simulink model "robotarm_A11"  (R2018b)
settings: Solver=FixedStepAuto  StartTime=0.0  StopTime=options.T_train  RelTol=1e-3  AbsTol=1e-6
undefined symbols (not defined in the file or in its folder): options
libraries: neural x132, simulink x2
(part 4 of 6)

== system robotarm_A11/NN/Layer 3/Delays 1 ==
  "p{3}" : Inport  PortDimensions=30
      mask Display: e = 0.06;c1 = [120 230 180]/255;c2 = ([120 230 180]+0)/(256+128);c3 = ([120 230 180]+128)/(256+128);patch([0 1 1 0],[0 0 1 1],c1);patch([0 1 1 1-e 1-e 0+e],[0 0 1 1-e 0+e 0+e],c2);patch([0 0 1 1-e 0+e 0+e],[0 1 1 1-e 1-e 0+e],c3);plot([0 1 1 0 0],[0 0 1 1 0]);
  mux : Mux  Inputs=1
      mask Display: e = 0.06;c1 = [120 150 230]/255;c2 = ([120 150 230]+0)/383;c3 = ([120 150 230]+128)/383;patch([0 1 1 0],[0 0 1 1],c1);patch([0 1 1 1-e 1-e 0+e],[0 0 1 1-e 0+e 0+e],c2);patch([0 0 1 1-e 0+e 0+e],[0 1 1 1-e 1-e 0+e],c3);plot([0 1 1 0 0],[0 0 1 1 0]);disp('Mux')
  "pd{3,2}" : Outport
      mask Display: e = 0.06;c1 = [120 230 180]/255;c2 = ([120 230 180]+0)/(256+128);c3 = ([120 230 180]+128)/(256+128);patch([0 1 1 0],[0 0 1 1],c1);patch([0 1 1 1-e 1-e 0+e],[0 0 1 1-e 0+e 0+e],c2);patch([0 0 1 1-e 0+e 0+e],[0 1 1 1-e 1-e 0+e],c3);plot([0 1 1 0 0],[0 0 1 1 0]);
  wires:
  "p{3}"/1 -> mux/1
  mux/1 -> "pd{3,2}"/1

== system robotarm_A11/NN/Layer 3/LW{3,2} ==
  "ad{3,2}" : Inport  PortDimensions=30
      mask Display: e = 0.06;c1 = [120 230 180]/255;c2 = ([120 230 180]+0)/(256+128);c3 = ([120 230 180]+128)/(256+128);patch([0 1 1 0],[0 0 1 1],c1);patch([0 1 1 1-e 1-e 0+e],[0 0 1 1-e 0+e 0+e],c2);patch([0 0 1 1-e 0+e 0+e],[0 1 1 1-e 1-e 0+e],c3);plot([0 1 1 0 0],[0 0 1 1 0]);
  "IW{3,2}(1,:)'" : Constant  Value=[0.07511090421461637245403863971660030074417591094970703125;-0.256099043433060113983401606674306094646453857421875;0.081996461567937439784969910760992206633090972900390625;-0.14973516379113960272917438487638719379901885986328125;0.5148961449988653793496951038832776248455047607421875;0.01324189378345717350848875781821334385313093662261962890625;0.2272209721687915850996120070703909732401371002197265625;-0.2208186824312869112052482023500488139688968658447265625;0.65756683071975541299281076135230250656604766845703125;-0.22237646509733133282082917503430508077144622802734375;-0.3308957162516181771394485622295178472995758056640625;0.637401045576047931007224178756587207317352294921875;0.667089213297717975592604489065706729888916015625;0.497075395905719308320414029367384500801563262939453125;-0.1445442468661915225158764997104299254715442657470703125;-0.336243110161506819633103759770165197551250457763671875;-0.65568518383315710362779782371944747865200042724609375;-0.6382390498773180542713134855148382484912872314453125;-0.44979178921980411676173616797314025461673736572265625;-0.2575443668624275428413739064126275479793548583984375;0.251838451386020290012623945585801266133785247802734375;0.84864546013635833165977828684845007956027984619140625;-0.31882372388745905400497804293991066515445709228515625;-0.27920298783133612463558392846607603132724761962890625;0.81251359569967795959399836647207848727703094482421875;-0.445650703236170731003085165866650640964508056640625;0.12363838330791576680667276377789676189422607421875;0.37180610815353876130728849602746777236461639404296875;-0.239048902638888172145215094133163802325725555419921875;0.06162269083689660142955091259864275343716144561767578125]
      mask Display: e = 0.06;c1 = [120 150 230]/255;c2 = ([120 150 230]+0)/383;c3 = ([120 150 230]+128)/383;patch([0 1 1 0],[0 0 1 1],c1);patch([0 1 1 1-e 1-e 0+e],[0 0 1 1-e 0+e 0+e],c2);patch([0 0 1 1-e 0+e 0+e],[0 1 1 1-e 1-e 0+e],c3);plot([0 1 1 0 0],[0 0 1 1 0]);disp('weights');
  Mux : Mux  Inputs=1
      mask Display: e = 0.06;c1 = [120 150 230]/255;c2 = ([120 150 230]+0)/383;c3 = ([120 150 230]+128)/383;patch([0 1 1 0],[0 0 1 1],c1);patch([0 1 1 1-e 1-e 0+e],[0 0 1 1-e 0+e 0+e],c2);patch([0 0 1 1-e 0+e 0+e],[0 1 1 1-e 1-e 0+e],c3);plot([0 1 1 0 0],[0 0 1 1 0]);disp('Mux');
  dotprod1 : neural/Weight Functions/dotprod
  "lz{3,2}" : Outport
      mask Display: e = 0.06;c1 = [120 230 180]/255;c2 = ([120 230 180]+0)/(256+128);c3 = ([120 230 180]+128)/(256+128);patch([0 1 1 0],[0 0 1 1],c1);patch([0 1 1 1-e 1-e 0+e],[0 0 1 1-e 0+e 0+e],c2);patch([0 0 1 1-e 0+e 0+e],[0 1 1 1-e 1-e 0+e],c3);plot([0 1 1 0 0],[0 0 1 1 0]);
  wires:
  "IW{3,2}(1,:)'"/1 -> dotprod1/1
  "ad{3,2}"/1 -> dotprod1/2
  dotprod1/1 -> Mux/1
  Mux/1 -> "lz{3,2}"/1

== system robotarm_A11/NN_cex_1/Layer 1/Delays 1 ==
  "p{1}" : Inport  PortDimensions=10
      mask Display: e = 0.06;c1 = [120 230 180]/255;c2 = ([120 230 180]+0)/(256+128);c3 = ([120 230 180]+128)/(256+128);patch([0 1 1 0],[0 0 1 1],c1);patch([0 1 1 1-e 1-e 0+e],[0 0 1 1-e 0+e 0+e],c2);patch([0 0 1 1-e 0+e 0+e],[0 1 1 1-e 1-e 0+e],c3);plot([0 1 1 0 0],[0 0 1 1 0]);
  mux : Mux  Inputs=1
      mask Display: e = 0.06;c1 = [120 150 230]/255;c2 = ([120 150 230]+0)/383;c3 = ([120 150 230]+128)/383;patch([0 1 1 0],[0 0 1 1],c1);patch([0 1 1 1-e 1-e 0+e],[0 0 1 1-e 0+e 0+e],c2);patch([0 0 1 1-e 0+e 0+e],[0 1 1 1-e 1-e 0+e],c3);plot([0 1 1 0 0],[0 0 1 1 0]);disp('Mux')
  "pd{1,1}" : Outport
      mask Display: e = 0.06;c1 = [120 230 180]/255;c2 = ([120 230 180]+0)/(256+128);c3 = ([120 230 180]+128)/(256+128);patch([0 1 1 0],[0 0 1 1],c1);patch([0 1 1 1-e 1-e 0+e],[0 0 1 1-e 0+e 0+e],c2);patch([0 0 1 1-e 0+e 0+e],[0 1 1 1-e 1-e 0+e],c3);plot([0 1 1 0 0],[0 0 1 1 0]);
  wires:
  "p{1}"/1 -> mux/1
  mux/1 -> "pd{1,1}"/1

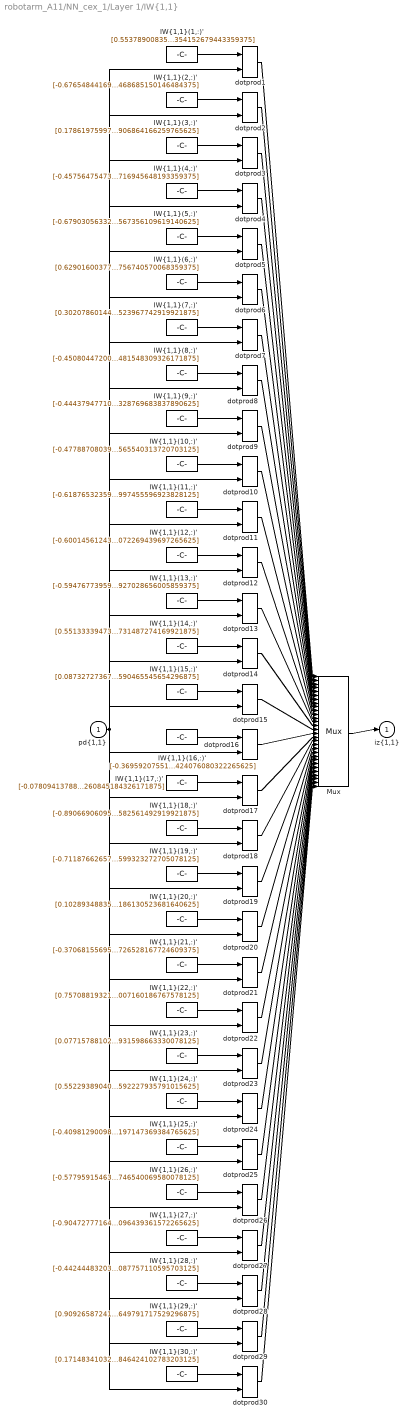
== system robotarm_A11/NN_cex_1/Layer 1/IW{1,1} ==
  "pd{1,1}" : Inport  PortDimensions=10
      mask Display: e = 0.06;c1 = [120 230 180]/255;c2 = ([120 230 180]+0)/(256+128);c3 = ([120 230 180]+128)/(256+128);patch([0 1 1 0],[0 0 1 1],c1);patch([0 1 1 1-e 1-e 0+e],[0 0 1 1-e 0+e 0+e],c2);patch([0 0 1 1-e 0+e 0+e],[0 1 1 1-e 1-e 0+e],c3);plot([0 1 1 0 0],[0 0 1 1 0]);
  "IW{1,1}(1,:)'" : Constant  Value=[0.55378900835415312275955557197448797523975372314453125;-0.40002833313486885202792109339497983455657958984375;0.51972210734784318741930064788903109729290008544921875;0.035441252661289439351843810754871810786426067352294921875;0.58851130139368124094545464686234481632709503173828125;0.373001312883801616759882335827569477260112762451171875;0.1968531470949289874372567510363296605646610260009765625;0.38544814076508793210251724303816445171833038330078125;0.52673681147124951085203292677761055529117584228515625;-0.76855654247942906120982797801843844354152679443359375]
      mask Display: e = 0.06;c1 = [120 150 230]/255;c2 = ([120 150 230]+0)/383;c3 = ([120 150 230]+128)/383;patch([0 1 1 0],[0 0 1 1],c1);patch([0 1 1 1-e 1-e 0+e],[0 0 1 1-e 0+e 0+e],c2);patch([0 0 1 1-e 0+e 0+e],[0 1 1 1-e 1-e 0+e],c3);plot([0 1 1 0 0],[0 0 1 1 0]);disp('Weights');
  "IW{1,1}(10,:)'" : Constant  Value=[-0.4778870803942767420124937416403554379940032958984375;0.6900752686105564581708904370316304266452789306640625;-0.98186484510186577967516541320946998894214630126953125;0.23336405361311773898336241472861729562282562255859375;-0.1824514456856282940133695547046954743564128875732421875;-0.32496417137077726611238404075265862047672271728515625;-0.2353568335365051333862851379308267496526241302490234375;-0.70434093877248338255725457202061079442501068115234375;-0.822356843400018799883355313795618712902069091796875;-0.436132420338480042421025473231566138565540313720703125]
      mask Display: e = 0.06;c1 = [120 150 230]/255;c2 = ([120 150 230]+0)/383;c3 = ([120 150 230]+128)/383;patch([0 1 1 0],[0 0 1 1],c1);patch([0 1 1 1-e 1-e 0+e],[0 0 1 1-e 0+e 0+e],c2);patch([0 0 1 1-e 0+e 0+e],[0 1 1 1-e 1-e 0+e],c3);plot([0 1 1 0 0],[0 0 1 1 0]);disp('Weights');
  "IW{1,1}(11,:)'" : Constant  Value=[-0.61876532359386915427279518553405068814754486083984375;0.50689349511924053359734898549504578113555908203125;-0.649599651050624782300246806698851287364959716796875;0.7245121834552035178234064005664549767971038818359375;0.363381703915839182617020242105354554951190948486328125;0.4964562727736183678217685155686922371387481689453125;0.761855040645396552889678787323646247386932373046875;-0.36285385966649152944540901444270275533199310302734375;-0.293639375529885671145535752657451666891574859619140625;0.177344276871376493875942514932830817997455596923828125]
      mask Display: e = 0.06;c1 = [120 150 230]/255;c2 = ([120 150 230]+0)/383;c3 = ([120 150 230]+128)/383;patch([0 1 1 0],[0 0 1 1],c1);patch([0 1 1 1-e 1-e 0+e],[0 0 1 1-e 0+e 0+e],c2);patch([0 0 1 1-e 0+e 0+e],[0 1 1 1-e 1-e 0+e],c3);plot([0 1 1 0 0],[0 0 1 1 0]);disp('Weights');
  "IW{1,1}(12,:)'" : Constant  Value=[-0.6001456124336532749197203884250484406948089599609375;0.33013842349252964236683283161255531013011932373046875;0.37826487084740623156875471977400593459606170654296875;0.391034981769335654444574856825056485831737518310546875;-0.4009196735274860312614464419311843812465667724609375;-0.46326488823745248790686446227482520043849945068359375;-0.002113484382197219728360959578594702179543673992156982421875;-0.438970954767614218727800334818311966955661773681640625;-0.1287719378224301547408714441189658828079700469970703125;-0.393126543674640060999081470072269439697265625]
      mask Display: e = 0.06;c1 = [120 150 230]/255;c2 = ([120 150 230]+0)/383;c3 = ([120 150 230]+128)/383;patch([0 1 1 0],[0 0 1 1],c1);patch([0 1 1 1-e 1-e 0+e],[0 0 1 1-e 0+e 0+e],c2);patch([0 0 1 1-e 0+e 0+e],[0 1 1 1-e 1-e 0+e],c3);plot([0 1 1 0 0],[0 0 1 1 0]);disp('Weights');
  "IW{1,1}(13,:)'" : Constant  Value=[-0.59476773959747486486548950779251754283905029296875;0.68919297431726411762298312169150449335575103759765625;0.1486056477337203418631617068967898376286029815673828125;-0.470729441790507963094825072403182275593280792236328125;0.4541780356710631849637138657271862030029296875;0.61892264157389453860247385819093324244022369384765625;0.415136576615699970371764493393129669129848480224609375;0.552166667443289238548231878667138516902923583984375;-0.43205002994984964548308425946743227541446685791015625;-0.46954834181149107674713150117895565927028656005859375]
      mask Display: e = 0.06;c1 = [120 150 230]/255;c2 = ([120 150 230]+0)/383;c3 = ([120 150 230]+128)/383;patch([0 1 1 0],[0 0 1 1],c1);patch([0 1 1 1-e 1-e 0+e],[0 0 1 1-e 0+e 0+e],c2);patch([0 0 1 1-e 0+e 0+e],[0 1 1 1-e 1-e 0+e],c3);plot([0 1 1 0 0],[0 0 1 1 0]);disp('Weights');
  "IW{1,1}(14,:)'" : Constant  Value=[0.55133339473071252267999398100073449313640594482421875;-0.2147279854494033857204016157993464730679988861083984375;-0.2208693068614927812465253964546718634665012359619140625;-0.08136652886051672084466446221995283849537372589111328125;-0.3735482426604528338742738924338482320308685302734375;-0.753054203048517223351154825650155544281005859375;-0.7437151949203808509736290943692438304424285888671875;-0.281684848857854774895059790651430375874042510986328125;-0.74895187646671657066832494820118881762027740478515625;-1.04045419377120396120517398230731487274169921875]
      mask Display: e = 0.06;c1 = [120 150 230]/255;c2 = ([120 150 230]+0)/383;c3 = ([120 150 230]+128)/383;patch([0 1 1 0],[0 0 1 1],c1);patch([0 1 1 1-e 1-e 0+e],[0 0 1 1-e 0+e 0+e],c2);patch([0 0 1 1-e 0+e 0+e],[0 1 1 1-e 1-e 0+e],c3);plot([0 1 1 0 0],[0 0 1 1 0]);disp('Weights');
  "IW{1,1}(15,:)'" : Constant  Value=[0.08732727367047816990908160050821607001125812530517578125;0.7188956926522018786585022098734043538570404052734375;0.5767351719523496900166037448798306286334991455078125;0.022544738930116443864637432170638930983841419219970703125;0.242667792684291450111544463652535341680049896240234375;-1.079378327692382288915950994123704731464385986328125;0.27181981404487054465590745166991837322711944580078125;0.312466232474387928252923529726103879511356353759765625;0.0284706853528155189037018857334260246716439723968505859375;0.67191294556673486493281188813853077590465545654296875]
      mask Display: e = 0.06;c1 = [120 150 230]/255;c2 = ([120 150 230]+0)/383;c3 = ([120 150 230]+128)/383;patch([0 1 1 0],[0 0 1 1],c1);patch([0 1 1 1-e 1-e 0+e],[0 0 1 1-e 0+e 0+e],c2);patch([0 0 1 1-e 0+e 0+e],[0 1 1 1-e 1-e 0+e],c3);plot([0 1 1 0 0],[0 0 1 1 0]);disp('Weights');
  "IW{1,1}(16,:)'" : Constant  Value=[-0.369592075516808560298187558146310038864612579345703125;0.95996493439695196325800452541443519294261932373046875;-0.50046865585050592795113288957509212195873260498046875;-0.410874434876904948144016316291526891291141510009765625;0.489781456141347160126997550833038985729217529296875;-0.93775511796223354199497634908766485750675201416015625;0.84159793108069036460250345044187270104885101318359375;0.042470512506688894160955527468104264698922634124755859375;0.293743829330801398125316836740239523351192474365234375;-0.418429180149094526175446162596927024424076080322265625]
      mask Display: e = 0.06;c1 = [120 150 230]/255;c2 = ([120 150 230]+0)/383;c3 = ([120 150 230]+128)/383;patch([0 1 1 0],[0 0 1 1],c1);patch([0 1 1 1-e 1-e 0+e],[0 0 1 1-e 0+e 0+e],c2);patch([0 0 1 1-e 0+e 0+e],[0 1 1 1-e 1-e 0+e],c3);plot([0 1 1 0 0],[0 0 1 1 0]);disp('Weights');
  "IW{1,1}(17,:)'" : Constant  Value=[-0.07809413788814582868536007254078867845237255096435546875;0.38353705545048077940606390257016755640506744384765625;-0.0017825378952640697459430807469971114187501370906829833984375;0.32868529336038287969046223224722780287265777587890625;-0.324134166881641594404328543532756157219409942626953125;-0.11838753778584253095740308481254032813012599945068359375;0.56754476329094127873275965612265281379222869873046875;-0.8977738792393186173512731329537928104400634765625;0.76394804482473632756267534205107949674129486083984375;1.176816594973402185786426343838684260845184326171875]
      mask Display: e = 0.06;c1 = [120 150 230]/255;c2 = ([120 150 230]+0)/383;c3 = ([120 150 230]+128)/383;patch([0 1 1 0],[0 0 1 1],c1);patch([0 1 1 1-e 1-e 0+e],[0 0 1 1-e 0+e 0+e],c2);patch([0 0 1 1-e 0+e 0+e],[0 1 1 1-e 1-e 0+e],c3);plot([0 1 1 0 0],[0 0 1 1 0]);disp('Weights');
  "IW{1,1}(18,:)'" : Constant  Value=[-0.8906690609565892646770635110442526638507843017578125;0.52672100716129766073692053396371193230152130126953125;0.422594444721862971814374532186775468289852142333984375;0.165946743221597914352827274342416785657405853271484375;0.6079356672903697411669554639956913888454437255859375;0.231823589748013036970775146983214654028415679931640625;0.79964219274385450741959857623442076146602630615234375;0.6518402694446481238088608733960427343845367431640625;0.191187367219683046482003874189103953540325164794921875;0.5083414959308221181544240607763640582561492919921875]
      mask Display: e = 0.06;c1 = [120 150 230]/255;c2 = ([120 150 230]+0)/383;c3 = ([120 150 230]+128)/383;patch([0 1 1 0],[0 0 1 1],c1);patch([0 1 1 1-e 1-e 0+e],[0 0 1 1-e 0+e 0+e],c2);patch([0 0 1 1-e 0+e 0+e],[0 1 1 1-e 1-e 0+e],c3);plot([0 1 1 0 0],[0 0 1 1 0]);disp('Weights');
  "IW{1,1}(19,:)'" : Constant  Value=[-0.71187662657045513991960206112707965075969696044921875;-0.74947909587272298903570799666340462863445281982421875;0.49718937350948533282490870988112874329090118408203125;0.38179457175583497718918124519404955208301544189453125;-0.6592711061060170241177047500968910753726959228515625;-0.264773654756297827095323782486957497894763946533203125;0.21441882691139735328533788560889661312103271484375;0.2291619051115253158368290087310015223920345306396484375;-0.1418755385024787207814966905061737634241580963134765625;-0.72900230756988826374964673959766514599323272705078125]
      mask Display: e = 0.06;c1 = [120 150 230]/255;c2 = ([120 150 230]+0)/383;c3 = ([120 150 230]+128)/383;patch([0 1 1 0],[0 0 1 1],c1);patch([0 1 1 1-e 1-e 0+e],[0 0 1 1-e 0+e 0+e],c2);patch([0 0 1 1-e 0+e 0+e],[0 1 1 1-e 1-e 0+e],c3);plot([0 1 1 0 0],[0 0 1 1 0]);disp('Weights');
  "IW{1,1}(2,:)'" : Constant  Value=[-0.6765484416959617330888931974186562001705169677734375;-0.781602512745850130926328347413800656795501708984375;0.85203687921405701910515517738531343638896942138671875;0.5385632970055862500657894997857511043548583984375;-0.60509709896651509009046776554896496236324310302734375;-0.2440369063980442898564859888210776261985301971435546875;-0.67637725797926151471983757801353931427001953125;-0.333291868234093124900851989877992309629917144775390625;-0.0853850172003989549285307703030412085354328155517578125;0.66990325024174113277553033185540698468685150146484375]
      mask Display: e = 0.06;c1 = [120 150 230]/255;c2 = ([120 150 230]+0)/383;c3 = ([120 150 230]+128)/383;patch([0 1 1 0],[0 0 1 1],c1);patch([0 1 1 1-e 1-e 0+e],[0 0 1 1-e 0+e 0+e],c2);patch([0 0 1 1-e 0+e 0+e],[0 1 1 1-e 1-e 0+e],c3);plot([0 1 1 0 0],[0 0 1 1 0]);disp('Weights');
  "IW{1,1}(20,:)'" : Constant  Value=[0.10289348835353044619989049124342272989451885223388671875;-0.4864311718452249966304634654079563915729522705078125;0.55019384700719931036161369775072671473026275634765625;0.227872600688055815254529079538770020008087158203125;-0.11288364590610307225393427188464556820690631866455078125;-0.7437389524921449446281940254266373813152313232421875;-0.5171424950133698406062876529176719486713409423828125;0.339576636279000421136942122757318429648876190185546875;-0.275941271419780365103946451199590228497982025146484375;0.6563524507375293470801125295110978186130523681640625]
      mask Display: e = 0.06;c1 = [120 150 230]/255;c2 = ([120 150 230]+0)/383;c3 = ([120 150 230]+128)/383;patch([0 1 1 0],[0 0 1 1],c1);patch([0 1 1 1-e 1-e 0+e],[0 0 1 1-e 0+e 0+e],c2);patch([0 0 1 1-e 0+e 0+e],[0 1 1 1-e 1-e 0+e],c3);plot([0 1 1 0 0],[0 0 1 1 0]);disp('Weights');
  "IW{1,1}(21,:)'" : Constant  Value=[-0.370681556957689173348313715905533172190189361572265625;0.86476817585020082645996808423660695552825927734375;-0.499742084321956936410202843035222031176090240478515625;0.01799270699531167749807281097673694603145122528076171875;0.672613806095245791993875172920525074005126953125;-0.32812357901071831367545428292942233383655548095703125;0.04257078178206423479945641474841977469623088836669921875;-0.48553580142793661966749141356558538973331451416015625;0.22289096525600637921371571792406029999256134033203125;-0.389180074830056843548931055920547805726528167724609375]
      mask Display: e = 0.06;c1 = [120 150 230]/255;c2 = ([120 150 230]+0)/383;c3 = ([120 150 230]+128)/383;patch([0 1 1 0],[0 0 1 1],c1);patch([0 1 1 1-e 1-e 0+e],[0 0 1 1-e 0+e 0+e],c2);patch([0 0 1 1-e 0+e 0+e],[0 1 1 1-e 1-e 0+e],c3);plot([0 1 1 0 0],[0 0 1 1 0]);disp('Weights');
  "IW{1,1}(22,:)'" : Constant  Value=[0.75708819321521547696107745650806464254856109619140625;0.25672728337317696212238615771639160811901092529296875;-0.2293107925262417301492945398422307334840297698974609375;0.8093632559271741744311157162883318960666656494140625;0.344008895567533390380532409835723228752613067626953125;-0.350459432030607975772085183052695356309413909912109375;0.07772012143806479589347446790270623750984668731689453125;-0.565722173385986071281195108895190060138702392578125;-0.097736781313982612484636547378613613545894622802734375;0.277467687629263715098915099588339217007160186767578125]
      mask Display: e = 0.06;c1 = [120 150 230]/255;c2 = ([120 150 230]+0)/383;c3 = ([120 150 230]+128)/383;patch([0 1 1 0],[0 0 1 1],c1);patch([0 1 1 1-e 1-e 0+e],[0 0 1 1-e 0+e 0+e],c2);patch([0 0 1 1-e 0+e 0+e],[0 1 1 1-e 1-e 0+e],c3);plot([0 1 1 0 0],[0 0 1 1 0]);disp('Weights');
  "IW{1,1}(23,:)'" : Constant  Value=[0.0771578810202487586078490267027518711984157562255859375;-0.02875313885587423012868413252363097853958606719970703125;1.14991515525726395452466022106818854808807373046875;-0.5241091439519178774020247146836481988430023193359375;-0.17449880613388213390635428368113934993743896484375;-0.398052659269516440065928009062190540134906768798828125;-0.2156094760457863690472635198602802120149135589599609375;-0.28168685153915629104659501535934396088123321533203125;0.87378518154396556116836336514097638428211212158203125;-0.288082781885752148287593854547594673931598663330078125]
      mask Display: e = 0.06;c1 = [120 150 230]/255;c2 = ([120 150 230]+0)/383;c3 = ([120 150 230]+128)/383;patch([0 1 1 0],[0 0 1 1],c1);patch([0 1 1 1-e 1-e 0+e],[0 0 1 1-e 0+e 0+e],c2);patch([0 0 1 1-e 0+e 0+e],[0 1 1 1-e 1-e 0+e],c3);plot([0 1 1 0 0],[0 0 1 1 0]);disp('Weights');
  "IW{1,1}(24,:)'" : Constant  Value=[0.5522938904057836939642811557860113680362701416015625;-0.05521257555263124616740100236711441539227962493896484375;0.63361755969526978304884323733858764171600341796875;-0.415645070670815408586662442758097313344478607177734375;0.04924609291869662397456153257735422812402248382568359375;0.84404167186953482637790102671715430915355682373046875;-0.5465407517109672763666594619280658662319183349609375;0.292715142416185347684631778975017368793487548828125;0.5260300608140953126934391548275016248226165771484375;-0.5186968482680980319088348551304079592227935791015625]
      mask Display: e = 0.06;c1 = [120 150 230]/255;c2 = ([120 150 230]+0)/383;c3 = ([120 150 230]+128)/383;patch([0 1 1 0],[0 0 1 1],c1);patch([0 1 1 1-e 1-e 0+e],[0 0 1 1-e 0+e 0+e],c2);patch([0 0 1 1-e 0+e 0+e],[0 1 1 1-e 1-e 0+e],c3);plot([0 1 1 0 0],[0 0 1 1 0]);disp('Weights');
  "IW{1,1}(25,:)'" : Constant  Value=[-0.40981290098953382372570786174037493765354156494140625;0.778989809366317675909385798149742186069488525390625;-0.58729332039798387565809889565571211278438568115234375;-0.1806171643904537216229755358654074370861053466796875;0.67408840662152702538634230222669430077075958251953125;-1.0793292420261713093765365556464530527591705322265625;0.60879251904144038309851794110727496445178985595703125;0.5122935184472845460135204120888374745845794677734375;-0.5827458237786988792805686898645944893360137939453125;-0.382188041911361742197783541996614076197147369384765625]
      mask Display: e = 0.06;c1 = [120 150 230]/255;c2 = ([120 150 230]+0)/383;c3 = ([120 150 230]+128)/383;patch([0 1 1 0],[0 0 1 1],c1);patch([0 1 1 1-e 1-e 0+e],[0 0 1 1-e 0+e 0+e],c2);patch([0 0 1 1-e 0+e 0+e],[0 1 1 1-e 1-e 0+e],c3);plot([0 1 1 0 0],[0 0 1 1 0]);disp('Weights');
  "IW{1,1}(26,:)'" : Constant  Value=[-0.57795915463737213002559656160883605480194091796875;-0.95794800979862670953224323966423980891704559326171875;0.7285311334751563006051355841918848454952239990234375;-0.3452310343901949796219241761718876659870147705078125;0.39271559323735261148868858072091825306415557861328125;0.65143434650189391277308459393680095672607421875;-0.0764479253964400751186758498079143464565277099609375;0.326107587259240661037296149515896104276180267333984375;0.2447857414114559537754445273094461299479007720947265625;0.565468245958776538628853813861496746540069580078125]
      mask Display: e = 0.06;c1 = [120 150 230]/255;c2 = ([120 150 230]+0)/383;c3 = ([120 150 230]+128)/383;patch([0 1 1 0],[0 0 1 1],c1);patch([0 1 1 1-e 1-e 0+e],[0 0 1 1-e 0+e 0+e],c2);patch([0 0 1 1-e 0+e 0+e],[0 1 1 1-e 1-e 0+e],c3);plot([0 1 1 0 0],[0 0 1 1 0]);disp('Weights');
  "IW{1,1}(27,:)'" : Constant  Value=[-0.90472777164449846853955250480794347822666168212890625;-0.230681151890325841780082782861427403986454010009765625;-0.318283932609921382805850953445769846439361572265625;0.475527363748191600478776308591477572917938232421875;-0.00797702646116844708845672329289300250820815563201904296875;0.6296425255322504188626453469623811542987823486328125;0.814335198577441854439484814065508544445037841796875;-0.10773134999736903860689807288508745841681957244873046875;0.6657337075735345610638660218683071434497833251953125;0.08943841373085516244234582927674637176096439361572265625]
      mask Display: e = 0.06;c1 = [120 150 230]/255;c2 = ([120 150 230]+0)/383;c3 = ([120 150 230]+128)/383;patch([0 1 1 0],[0 0 1 1],c1);patch([0 1 1 1-e 1-e 0+e],[0 0 1 1-e 0+e 0+e],c2);patch([0 0 1 1-e 0+e 0+e],[0 1 1 1-e 1-e 0+e],c3);plot([0 1 1 0 0],[0 0 1 1 0]);disp('Weights');
  "IW{1,1}(28,:)'" : Constant  Value=[-0.442444832037940327662539630182436667382717132568359375;0.584016083154378140562812404823489487171173095703125;0.24420740671438967428485966593143530189990997314453125;-0.674290581319769710688660779851488769054412841796875;-0.689991219470693639692626675241626799106597900390625;0.68799772923881830077874610651633702218532562255859375;-0.44476050168300307330326859300839714705944061279296875;0.989125187222113400054013254703022539615631103515625;0.36262574243727441203333228258998133242130279541015625;0.362599566330838396499558484720182605087757110595703125]
      mask Display: e = 0.06;c1 = [120 150 230]/255;c2 = ([120 150 230]+0)/383;c3 = ([120 150 230]+128)/383;patch([0 1 1 0],[0 0 1 1],c1);patch([0 1 1 1-e 1-e 0+e],[0 0 1 1-e 0+e 0+e],c2);patch([0 0 1 1-e 0+e 0+e],[0 1 1 1-e 1-e 0+e],c3);plot([0 1 1 0 0],[0 0 1 1 0]);disp('Weights');
  "IW{1,1}(29,:)'" : Constant  Value=[0.90926587241069045663977021831669844686985015869140625;-0.691860013044337751608736652997322380542755126953125;-0.441495608367609870814618489021086134016513824462890625;0.253939910762159881674193684375495649874210357666015625;-0.85963910611840310682651988827274180948734283447265625;0.64694819938157877015072472204337827861309051513671875;0.342735737417841967999976304781739600002765655517578125;0.4054784402841844492826339774182997643947601318359375;0.996792830303312005213456359342671930789947509765625;-0.02526429197925761371834596502594649791717529296875]
      mask Display: e = 0.06;c1 = [120 150 230]/255;c2 = ([120 150 230]+0)/383;c3 = ([120 150 230]+128)/383;patch([0 1 1 0],[0 0 1 1],c1);patch([0 1 1 1-e 1-e 0+e],[0 0 1 1-e 0+e 0+e],c2);patch([0 0 1 1-e 0+e 0+e],[0 1 1 1-e 1-e 0+e],c3);plot([0 1 1 0 0],[0 0 1 1 0]);disp('Weights');
  "IW{1,1}(3,:)'" : Constant  Value=[0.1786197599739836328058828485154663212597370147705078125;-1.0059263954570238919217217699042521417140960693359375;0.8004307589568504521793101957882754504680633544921875;-0.11655263292852023615520096200270927511155605316162109375;0.6004504260257819137081014559953473508358001708984375;-0.30003585769335117117151412458042614161968231201171875;0.412750284658198907106196884342352859675884246826171875;-0.367996152642487917017177778689074330031871795654296875;0.35353982596313515696095919338404200971126556396484375;1.007071414597183522943169009522534906864166259765625]
      mask Display: e = 0.06;c1 = [120 150 230]/255;c2 = ([120 150 230]+0)/383;c3 = ([120 150 230]+128)/383;patch([0 1 1 0],[0 0 1 1],c1);patch([0 1 1 1-e 1-e 0+e],[0 0 1 1-e 0+e 0+e],c2);patch([0 0 1 1-e 0+e 0+e],[0 1 1 1-e 1-e 0+e],c3);plot([0 1 1 0 0],[0 0 1 1 0]);disp('Weights');
  "IW{1,1}(30,:)'" : Constant  Value=[0.1714834103232745488032406910861027427017688751220703125;0.9043493859342086604868882204755209386348724365234375;-0.842611754852075289790036549675278365612030029296875;0.70987068509282080785993684912682510912418365478515625;-0.75782155959692076852007858178694732487201690673828125;0.11675023976314365115047877452525426633656024932861328125;-0.6979489928386086727840620369534008204936981201171875;-0.2088570850528912170585016383483889512717723846435546875;0.082515301009249586439153745232033543288707733154296875;-0.012134570601365475550625916412172955460846424102783203125]
      mask Display: e = 0.06;c1 = [120 150 230]/255;c2 = ([120 150 230]+0)/383;c3 = ([120 150 230]+128)/383;patch([0 1 1 0],[0 0 1 1],c1);patch([0 1 1 1-e 1-e 0+e],[0 0 1 1-e 0+e 0+e],c2);patch([0 0 1 1-e 0+e 0+e],[0 1 1 1-e 1-e 0+e],c3);plot([0 1 1 0 0],[0 0 1 1 0]);disp('Weights');
  "IW{1,1}(4,:)'" : Constant  Value=[-0.45756475473305346923780234646983444690704345703125;0.7100732302891012981405083337449468672275543212890625;-0.5905529550747867784110667344066314399242401123046875;0.1916870396182032421084073803285718895494937896728515625;0.85891573589324654580678952697780914604663848876953125;-0.098323413263364189962345562889822758734226226806640625;-0.01081946784307483318265941107938488130457699298858642578125;-0.82778781025502568002849557160516269505023956298828125;0.64805294011171332702048175633535720407962799072265625;-0.372167657243175964421055823549977503716945648193359375]
      mask Display: e = 0.06;c1 = [120 150 230]/255;c2 = ([120 150 230]+0)/383;c3 = ([120 150 230]+128)/383;patch([0 1 1 0],[0 0 1 1],c1);patch([0 1 1 1-e 1-e 0+e],[0 0 1 1-e 0+e 0+e],c2);patch([0 0 1 1-e 0+e 0+e],[0 1 1 1-e 1-e 0+e],c3);plot([0 1 1 0 0],[0 0 1 1 0]);disp('Weights');
  "IW{1,1}(5,:)'" : Constant  Value=[-0.67903056332520506099825752244214527308940887451171875;-0.71226188251845978793852509625139646232128143310546875;-0.29550337477607102609766798195778392255306243896484375;-0.5621706921562765746358536489424295723438262939453125;-0.360153407061320984805519174187793396413326263427734375;-0.085248687145863810687984596370370127260684967041015625;-0.89444245935023192206614339738734997808933258056640625;-0.2219122262053243588297846144996583461761474609375;0.63277175118875927939399161914479918777942657470703125;0.1775825484859347158650422215941944159567356109619140625]
      mask Display: e = 0.06;c1 = [120 150 230]/255;c2 = ([120 150 230]+0)/383;c3 = ([120 150 230]+128)/383;patch([0 1 1 0],[0 0 1 1],c1);patch([0 1 1 1-e 1-e 0+e],[0 0 1 1-e 0+e 0+e],c2);patch([0 0 1 1-e 0+e 0+e],[0 1 1 1-e 1-e 0+e],c3);plot([0 1 1 0 0],[0 0 1 1 0]);disp('Weights');
  "IW{1,1}(6,:)'" : Constant  Value=[0.62901600377946353948033220149227418005466461181640625;0.75670709546064696127132265246473252773284912109375;-0.95369060769107549813128343885182403028011322021484375;0.275443333114418764662190142189501784741878509521484375;0.409877180076590075241682598061743192374706268310546875;-0.47550323891740708948105975650832988321781158447265625;-0.274045478551425192303980793440132401883602142333984375;-0.06277228986576367797400877179825329221785068511962890625;-0.312588213170752859948464674744172953069210052490234375;0.443965158713444052462904210187844000756740570068359375]
      mask Display: e = 0.06;c1 = [120 150 230]/255;c2 = ([120 150 230]+0)/383;c3 = ([120 150 230]+128)/383;patch([0 1 1 0],[0 0 1 1],c1);patch([0 1 1 1-e 1-e 0+e],[0 0 1 1-e 0+e 0+e],c2);patch([0 0 1 1-e 0+e 0+e],[0 1 1 1-e 1-e 0+e],c3);plot([0 1 1 0 0],[0 0 1 1 0]);disp('Weights');
  "IW{1,1}(7,:)'" : Constant  Value=[0.30207860144034726079809161092271097004413604736328125;-0.93476265001382896624448903821757994592189788818359375;0.8387386407380084119012053633923642337322235107421875;0.080057400288016056233431072541861794888973236083984375;-0.1984941934189104750796417420133366249501705169677734375;-0.469675665683895904312095126442727632820606231689453125;0.74592304698054834322107353727915324270725250244140625;0.79319134172268501714597732643596827983856201171875;-0.1552804694120588357986179062208975665271282196044921875;0.367640351385918939808306049599195830523967742919921875]
      mask Display: e = 0.06;c1 = [120 150 230]/255;c2 = ([120 150 230]+0)/383;c3 = ([120 150 230]+128)/383;patch([0 1 1 0],[0 0 1 1],c1);patch([0 1 1 1-e 1-e 0+e],[0 0 1 1-e 0+e 0+e],c2);patch([0 0 1 1-e 0+e 0+e],[0 1 1 1-e 1-e 0+e],c3);plot([0 1 1 0 0],[0 0 1 1 0]);disp('Weights');
  "IW{1,1}(8,:)'" : Constant  Value=[-0.45080447200377171679264165504719130694866180419921875;0.471262137454936780311953725686180405318737030029296875;0.11563623433188284506112353255957714281976222991943359375;0.341385674410052242233604147259029559791088104248046875;0.561635959332757561668358903261832892894744873046875;-0.8920735471324332532816470120451413094997406005859375;-0.53591301120284040582220086434972472488880157470703125;0.44217298383291037122688749150256626307964324951171875;-0.388630772163258197959834205903462134301662445068359375;-0.244344517832601137996562101761810481548309326171875]
      mask Display: e = 0.06;c1 = [120 150 230]/255;c2 = ([120 150 230]+0)/383;c3 = ([120 150 230]+128)/383;patch([0 1 1 0],[0 0 1 1],c1);patch([0 1 1 1-e 1-e 0+e],[0 0 1 1-e 0+e 0+e],c2);patch([0 0 1 1-e 0+e 0+e],[0 1 1 1-e 1-e 0+e],c3);plot([0 1 1 0 0],[0 0 1 1 0]);disp('Weights');
  "IW{1,1}(9,:)'" : Constant  Value=[-0.444379477103415576610956350123160518705844879150390625;0.4922119252336418782078908407129347324371337890625;-0.054896579343914730930720224932883866131305694580078125;-0.0963702177642190294104551639975397847592830657958984375;0.141036843203443285066356338575133122503757476806640625;-1.08303526424540574879529231111519038677215576171875;0.769436001251385004451321947271935641765594482421875;0.36921707280765303504921348576317541301250457763671875;-0.54983487682726550627165806872653774917125701904296875;-0.91933536794139403269809918128885328769683837890625]
      mask Display: e = 0.06;c1 = [120 150 230]/255;c2 = ([120 150 230]+0)/383;c3 = ([120 150 230]+128)/383;patch([0 1 1 0],[0 0 1 1],c1);patch([0 1 1 1-e 1-e 0+e],[0 0 1 1-e 0+e 0+e],c2);patch([0 0 1 1-e 0+e 0+e],[0 1 1 1-e 1-e 0+e],c3);plot([0 1 1 0 0],[0 0 1 1 0]);disp('Weights');
  Mux : Mux  Inputs=30
      mask Display: e = 0.06;c1 = [120 150 230]/255;c2 = ([120 150 230]+0)/383;c3 = ([120 150 230]+128)/383;patch([0 1 1 0],[0 0 1 1],c1);patch([0 1 1 1-e 1-e 0+e],[0 0 1 1-e 0+e 0+e],c2);patch([0 0 1 1-e 0+e 0+e],[0 1 1 1-e 1-e 0+e],c3);plot([0 1 1 0 0],[0 0 1 1 0]);disp('Mux');
  dotprod{1..30} (30 alike) : neural/Weight Functions/dotprod
  "iz{1,1}" : Outport
      mask Display: e = 0.06;c1 = [120 230 180]/255;c2 = ([120 230 180]+0)/(256+128);c3 = ([120 230 180]+128)/(256+128);patch([0 1 1 0],[0 0 1 1],c1);patch([0 1 1 1-e 1-e 0+e],[0 0 1 1-e 0+e 0+e],c2);patch([0 0 1 1-e 0+e 0+e],[0 1 1 1-e 1-e 0+e],c3);plot([0 1 1 0 0],[0 0 1 1 0]);
  wires:
  "IW{1,1}(1,:)'"/1 -> dotprod1/1
  "pd{1,1}"/1 -> dotprod1/2, dotprod2/2, dotprod3/2, dotprod4/2, dotprod5/2, dotprod6/2, dotprod7/2, dotprod8/2, dotprod9/2, dotprod10/2, dotprod11/2, dotprod12/2, dotprod13/2, dotprod14/2, dotprod15/2, dotprod16/2, dotprod17/2, dotprod18/2, dotprod19/2, dotprod20/2, dotprod21/2, dotprod22/2, dotprod23/2, dotprod24/2, dotprod25/2, dotprod26/2, dotprod27/2, dotprod28/2, dotprod29/2, dotprod30/2
  dotprod1/1 -> Mux/1
  "IW{1,1}(2,:)'"/1 -> dotprod2/1
  dotprod2/1 -> Mux/2
  "IW{1,1}(3,:)'"/1 -> dotprod3/1
  dotprod3/1 -> Mux/3
  "IW{1,1}(4,:)'"/1 -> dotprod4/1
  dotprod4/1 -> Mux/4
  "IW{1,1}(5,:)'"/1 -> dotprod5/1
  dotprod5/1 -> Mux/5
  "IW{1,1}(6,:)'"/1 -> dotprod6/1
  dotprod6/1 -> Mux/6
  "IW{1,1}(7,:)'"/1 -> dotprod7/1
  dotprod7/1 -> Mux/7
  "IW{1,1}(8,:)'"/1 -> dotprod8/1
  dotprod8/1 -> Mux/8
  "IW{1,1}(9,:)'"/1 -> dotprod9/1
  dotprod9/1 -> Mux/9
  "IW{1,1}(10,:)'"/1 -> dotprod10/1
  dotprod10/1 -> Mux/10
  "IW{1,1}(11,:)'"/1 -> dotprod11/1
  dotprod11/1 -> Mux/11
  "IW{1,1}(12,:)'"/1 -> dotprod12/1
  dotprod12/1 -> Mux/12
  "IW{1,1}(13,:)'"/1 -> dotprod13/1
  dotprod13/1 -> Mux/13
  "IW{1,1}(14,:)'"/1 -> dotprod14/1
  dotprod14/1 -> Mux/14
  "IW{1,1}(15,:)'"/1 -> dotprod15/1
  dotprod15/1 -> Mux/15
  "IW{1,1}(16,:)'"/1 -> dotprod16/1
  dotprod16/1 -> Mux/16
  "IW{1,1}(17,:)'"/1 -> dotprod17/1
  dotprod17/1 -> Mux/17
  "IW{1,1}(18,:)'"/1 -> dotprod18/1
  dotprod18/1 -> Mux/18
  "IW{1,1}(19,:)'"/1 -> dotprod19/1
  dotprod19/1 -> Mux/19
  "IW{1,1}(20,:)'"/1 -> dotprod20/1
  dotprod20/1 -> Mux/20
  "IW{1,1}(21,:)'"/1 -> dotprod21/1
  dotprod21/1 -> Mux/21
  "IW{1,1}(22,:)'"/1 -> dotprod22/1
  dotprod22/1 -> Mux/22
  "IW{1,1}(23,:)'"/1 -> dotprod23/1
  dotprod23/1 -> Mux/23
  "IW{1,1}(24,:)'"/1 -> dotprod24/1
  dotprod24/1 -> Mux/24
  "IW{1,1}(25,:)'"/1 -> dotprod25/1
  dotprod25/1 -> Mux/25
  "IW{1,1}(26,:)'"/1 -> dotprod26/1
  dotprod26/1 -> Mux/26
  "IW{1,1}(27,:)'"/1 -> dotprod27/1
  dotprod27/1 -> Mux/27
  "IW{1,1}(28,:)'"/1 -> dotprod28/1
  dotprod28/1 -> Mux/28
  "IW{1,1}(29,:)'"/1 -> dotprod29/1
  dotprod29/1 -> Mux/29
  "IW{1,1}(30,:)'"/1 -> dotprod30/1
  dotprod30/1 -> Mux/30
  Mux/1 -> "iz{1,1}"/1

== system robotarm_A11/NN_cex_1/Layer 2/Delays 1 ==
  "p{2}" : Inport  PortDimensions=30
      mask Display: e = 0.06;c1 = [120 230 180]/255;c2 = ([120 230 180]+0)/(256+128);c3 = ([120 230 180]+128)/(256+128);patch([0 1 1 0],[0 0 1 1],c1);patch([0 1 1 1-e 1-e 0+e],[0 0 1 1-e 0+e 0+e],c2);patch([0 0 1 1-e 0+e 0+e],[0 1 1 1-e 1-e 0+e],c3);plot([0 1 1 0 0],[0 0 1 1 0]);
  mux : Mux  Inputs=1
      mask Display: e = 0.06;c1 = [120 150 230]/255;c2 = ([120 150 230]+0)/383;c3 = ([120 150 230]+128)/383;patch([0 1 1 0],[0 0 1 1],c1);patch([0 1 1 1-e 1-e 0+e],[0 0 1 1-e 0+e 0+e],c2);patch([0 0 1 1-e 0+e 0+e],[0 1 1 1-e 1-e 0+e],c3);plot([0 1 1 0 0],[0 0 1 1 0]);disp('Mux')
  "pd{2,1}" : Outport
      mask Display: e = 0.06;c1 = [120 230 180]/255;c2 = ([120 230 180]+0)/(256+128);c3 = ([120 230 180]+128)/(256+128);patch([0 1 1 0],[0 0 1 1],c1);patch([0 1 1 1-e 1-e 0+e],[0 0 1 1-e 0+e 0+e],c2);patch([0 0 1 1-e 0+e 0+e],[0 1 1 1-e 1-e 0+e],c3);plot([0 1 1 0 0],[0 0 1 1 0]);
  wires:
  "p{2}"/1 -> mux/1
  mux/1 -> "pd{2,1}"/1
